simulink subsystem "serial_to_parallel"  (R2022b)
settings: Solver=VariableStepAuto  StartTime=0.0  StopTime=10.0  RelTol=1e-3
settings Model: Creator=Ali-Laptop  LastModifiedBy=Ali-Laptop

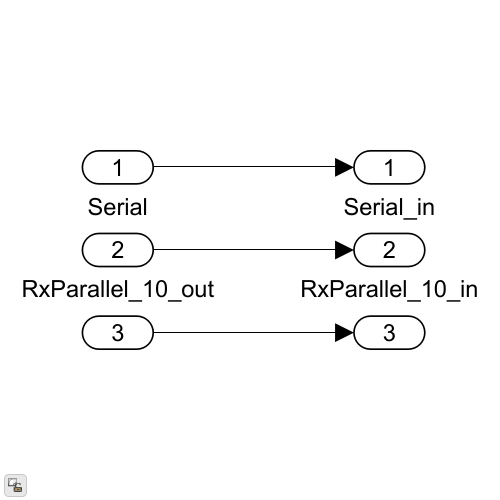
[thumbnail: Simulink's stored preview of the top-level diagram]
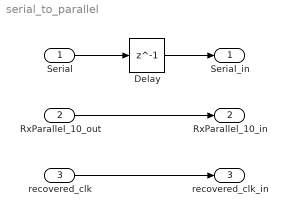
== system serial_to_parallel ==
  Serial : Inport
  RxParallel_10_out : Inport  Port=2
  recovered_clk : Inport  Port=3
  Delay : Delay  DelayLength=1
  Serial_in : Outport
  RxParallel_10_in : Outport  Port=2
  recovered_clk_in : Outport  Port=3
  wires:
  RxParallel_10_out/1 -> RxParallel_10_in/1
  Serial/1 -> Delay/1
  recovered_clk/1 -> recovered_clk_in/1
  Delay/1 -> Serial_in/1
